simulink model "gm_Approximate_id_46f54147700b843c92a4e9dfa9c6267fbdad2df7"  (R2020a)
settings: Solver=VariableStepAuto  StartTime=0.0  StopTime=10.0  RelTol=1e-3
model workspace (MAT data in the model file):
  InputValues_20210723T014030585 = [-8 -7.99975585938 -7.99951171875 -7.99926757812 -7.9990234375 -7.99877929688 -7.99853515625 -7.99829101562 -7.998046875 -7.99780273438 -7.99755859375 -7.99731445312 ... (65536 elements, 65536x1)]
(part 2 of 2)

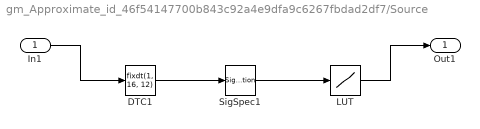
== system gm_Approximate_id_46f54147700b843c92a4e9dfa9c6267fbdad2df7/Source ==
  In1 : Inport  OutDataTypeStr=fixdt(1, 16, 12)  PortDimensions=1  SampleTime=0
  DTC1 : DataTypeConversion  OutDataTypeStr=fixdt(1, 16, 12)  RndMeth=Nearest  SampleTime=0
  LUT : Lookup_n-D  NumberOfTableDimensions=1  BreakpointsForDimension1="fi(\"numerictype\",numerictype(1,16,12),\"fimath\",fimath(\"RoundingMethod\", \"Floor\",\"OverflowAction\", \"Wrap\",\"ProductMode\",\"FullPrecision\",\"SumMode\",\"FullPrecision\"),\"Value\",\"[-8 -7.666748046875 -7.33349609375 -7.000244140625 -6.6669921875 -6.333740234375 -6.00048828125 -5.667236328125 -5.333984375 -5.000732421875 -4.66748046875 -4.334228515625 -4.0009765625 -3.667724609375 -3.33447265625 -3.001220703125 -2.66796875 -2.334716796875 -2.00146484375 -1.668212890625 -1.3349609375 -1.001708984375 -0.66845703125 -0.335205078125 -0.001953125 0.331298828125 0.66455078125 0.997802734375 1.3310546875 1.664306640625 1.99755859375 2.330810546875 2.6640625 2.997314453125 3.33056640625 3.663818359375 3.9970703125 4.330322265625 4.66357421875 4.996826171875 5.330078125 5.663330078125 5.99658203125 6.329833984375 6.6630859375 6.996337890625 7.32958984375 7.662841796875 7.99609375]\")"  Table="reshape(fi(\"numerictype\",numerictype(1,16,15),\"fimath\",fimath(\"RoundingMethod\", \"Floor\",\"OverflowAction\", \"Wrap\",\"ProductMode\",\"FullPrecision\",\"SumMode\",\"FullPrecision\"),\"Value\",\"[-1;-1;-1;-1;-1;-1;-1;-1;-1;-1;-1;-1;-0.99957275390625;-0.999481201171875;-0.996246337890625;-0.995147705078125;-0.990509033203125;-0.982269287109375;-0.9644775390625;-0.9324951171875;-0.8736572265625;-0.76776123046875;-0.590240478515625;-0.328399658203125;-0.000732421875;0.32513427734375;0.58795166015625;0.766754150390625;0.873870849609375;0.933197021484375;0.96527099609375;0.9818115234375;0.99041748046875;0.994659423828125;0.997589111328125;0.999969482421875;0.999359130859375;0.999969482421875;0.999969482421875;0.999969482421875;0.999969482421875;0.999969482421875;0.999969482421875;0.999969482421875;0.999969482421875;0.999969482421875;0.999969482421875;0.999969482421875;0.999969482421875]\"), [1  49])"  ExtrapMethod=Clip  SampleTime=0  OutDataTypeStr=fixdt(1, 16, 15)  RndMeth=Simplest  InputSameDT=on
  SigSpec1 : SignalSpecification  OutDataTypeStr=fixdt(1, 16, 12)  Dimensions=1
  Out1 : Outport
  wires:
  In1/1 -> DTC1/1
  DTC1/1 -> SigSpec1/1
  LUT/1 -> Out1/1
  SigSpec1/1 -> LUT/1
